simulink model "Panning"  (R2020b)
settings: Solver=VariableStepAuto  StartTime=0.0  StopTime=10  RelTol=1e-3
libraries: dspsrcs4 x1, dspvision x1, dspsnks4 x1
settings Model: Creator=JonathanPC  LastModifiedBy=JonathanPC

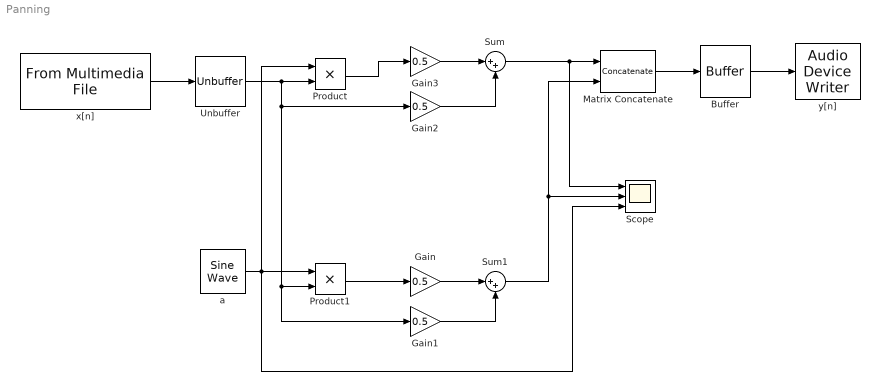
== system Panning ==
  Buffer : Buffer  OutputFrames=off
  Gain{,1..3} (4 alike) : Gain  Gain=0.5
  Matrix Concatenate : Concatenate  Mode=Multidimensional array  ConcatenateDimension=2
  Product : Product
  Product1 : Product
  Scope : Scope  NumInputPorts=3
  Sum : Sum  Inputs=|++
  Sum1 : Sum  Inputs=|++
  Unbuffer : Unbuffer
  a : dspsrcs4/Sine Wave  Amplitude=1  Frequency=0.2  Phase=0  SampleMode=Discrete  OutComplex=Real  CompMethod=Trigonometric fcn  TableSize=Speed  SampleTime=0.01  SamplesPerFrame=3  ResetState=Restart at time zero  OutputFrames=off  dataType=double  wordLen=16  udDataType=sfix(16)  fracBitsMode=Best precision  numFracBits=15  OutDataTypeStr=double  LastOutDataTypeStr=double
  x[n] : dspvision/From Multimedia File  inputFilename=C:\Users\JonathanPC\Documents\MATLAB\taller2\Sonido.wav  readRange=[1 Inf]  loop=on  numPlays=inf  outputStreams=Audio only  videoDataType=single  audioDataType=double  inheritSampleTime=on  userDefinedSampleTime=1/30  noAudioOutput=off  isIntensityVideo=off  fourcc=RGB  colorVideoFormat=Separate color signals  outputEOF=off  dataOrg=Column-major  audioFrameSize=1024  computeAudioFrameSize=off  outSamplingMode=Sample based
  y[n] : dspsnks4/Audio Device Writer  Driver=DirectSound  Device=Default  InheritSampleRate=on  SampleRate=44100  BitDepth=16-bit integer  BufferSize=4096  NumBuffers=10  DefaultOutputChannelMapping=on  OutputChannelMapping=1:2  OutputNumUnderrunSamples=off  DriverIdx=1  DeviceWarnFlag=''
  wires:
  Buffer/1 -> y[n]/1
  Sum1/1 -> Matrix Concatenate/2, Scope/2
  Product1/1 -> Gain/1
  Gain2/1 -> Sum/2
  Product/1 -> Gain3/1
  Gain/1 -> Sum1/1
  Sum/1 -> Scope/1, Matrix Concatenate/1
  Matrix Concatenate/1 -> Buffer/1
  Gain1/1 -> Sum1/2
  Unbuffer/1 -> Product/2, Gain1/1, Product1/2, Gain2/1
  a/1 -> Product/1, Scope/3, Product1/1
  x[n]/1 -> Unbuffer/1
  Gain3/1 -> Sum/1
